simulink model "VirtualMotoTemplate"  (R2025b)
settings: Solver=daessc  StartTime=0  StopTime=2474  FixedStep=.001  RelTol=1e-2  EnableMultiTasking=on
StopFcn:
  | %toc
undefined symbols (not defined in the file): AccelOvrCmd, CtrlTcuInitGear, DecelOvrCmd, Disabled, DriverPreviewDist, EnblAccelOvr, EnblDecelCmd, EnblSteerCmd, EnvAbsPrs, EnvAirTemp, EnvGrvty, EnvNomFrictionScaling, EnvNominalGrade, EnvWindVelX, EnvWindVelY, EnvWindVelZ, FTP75, MotoFrmInert, MotoFrmLngth, MotoFrmMass, MotoLowrFrntFrkMass, MotoRearArmLngth, MotoRearArmMass, MotoUpprFrntFrkMass, RiderLkAhdPtDstGain, RiderMass, ScnAccTbl, ScnBrkTbl, ScnCRMaxLatAccel, ScnCRRadius, ScnDLCGateLongPos, ScnDLCLatRef, ScnDLCLatRefOffset, ScnDLCLongRefBpt, ScnDLCLongRefStartPos, ScnDLCVehicleWidth, ScnFHCounterDwellTime, ScnFHInitialDwellTime, ScnFHReturnTime, ScnFHRollRateZeroCross, ScnFHSteerAmp, ScnFHSteerSpeed, ScnISHandwheelRate, ScnISMaxHandwheelAng, ScnISMaxLatAccel, ScnISSteerHoldTime, ScnLongPosBpts, ScnLongVelRef, ScnOvalTrackl, ScnOvalTrackpdst, ScnOvalTrackr, ScnSDDwellTime, ScnSDSteerAmp, ScnSDSteerFreq, ScnSSFinalFreq, ScnSSSteerAmp, ScnSSSweepTime, ScnStartTime, ScnStrgAngTbl, ScnStrgTrqTbl ... (+10)
libraries: simulink x16, vehdynlibscenariocommon x9, sm_lib x6, autolibshared x4, nesl_utility x4, vehdynlibviscommon x3, sim3dgroundtruthsensorlib x2, vehdynlibdriver x2, sharedtransform x1, autolibutils x1, sim3dautolib x1, sim3dlib x1
(part 2 of 6)

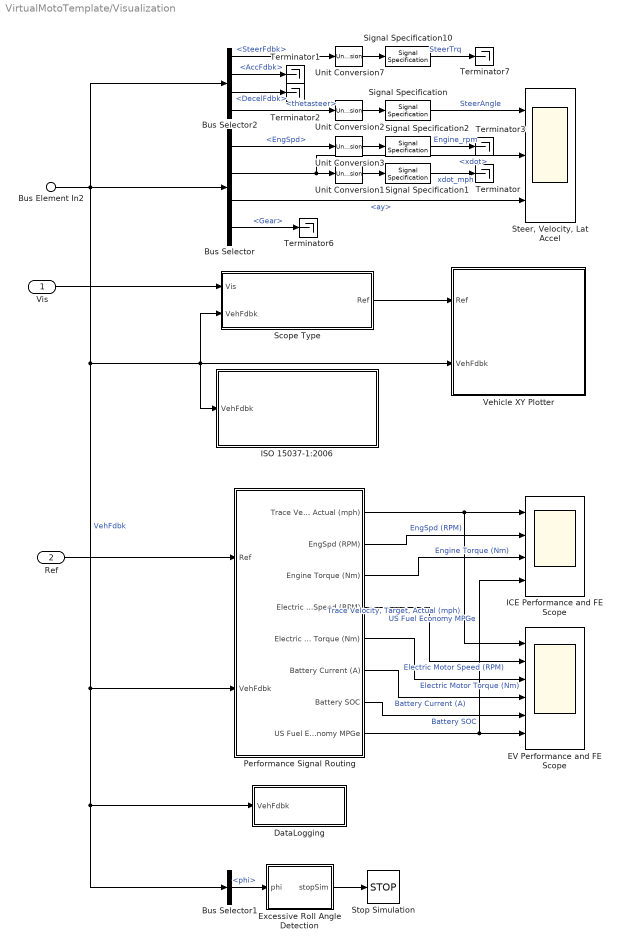
== system VirtualMotoTemplate/Visualization ==
  Vis : Inport
  Ref : Inport  Port=2
  Bus Element In2 : Inport  Port=3  PortName=VehFdbk
  Bus Selector : BusSelector  OutputSignals=Driveline.EngSpd,Body.BdyFrm.Cg.Vel.xdot,Body.BdyFrm.Cg.Acc.ay,Driveline.Gear
  Bus Selector1 : BusSelector  OutputSignals=Body.InertFrm.Cg.Ang.phi
  Bus Selector2 : BusSelector  OutputSignals=Rider.SteerFdbk,Rider.AccFdbk,Rider.DecelFdbk,Steer.Genrl.Ang.thetasteer
  DataLogging : Subsystem
  EV Performance and FE Scope : Scope  NumInputPorts=6
      settings: SampleTime=0.1  ActiveDisplayYMinimum=-0.55336  ActiveDisplayYMaximum=25.23635
  Excessive Roll Angle Detection : MATLAB Function  TreatAsAtomicUnit=on  SystemSampleTime=.1
  ICE Performance and FE Scope : Scope  NumInputPorts=4
      settings: SampleTime=0.1  ActiveDisplayYMinimum=-3.00968  ActiveDisplayYMaximum=25.77885
  ISO 15037-1:2006 : Subsystem  StopFcn=|  Variant=on  VariantControlMode=label  LabelModeActiveChoice=0  mask(ISO 15037-1:2006){Measurement=Disabled}
      | switch get_param(gcb,'Measurement')
      |     case 'Enabled'
      |        p=slproject.getCurrentProject;
      |        projectRoot=p.RootFolder;
      |        SySFolder=fullfile(projectRoot, 'System');
      |        Simulink.sdi.loadView([SySFolder filesep 'ISO15037_1_2006E.mldatx']);
      |        Simulink.sdi.view;
      | end
      mask prompts: Measurement "ISO Measurements"
      mask help: Enables display of ISO 15037-1:2006 standard measurement signals in the Simulation Data Inspector.
      mask init:
      | switch get_param(gcb,'Measurement')
      |     case 'Disabled'
      |         set_param(gcb,'OverrideUsingVariant','0')
      |     case 'Enabled'
      |        set_param(gcb,'OverrideUsingVariant','1')
      |     otherwise
      |        set_param(gcb,'OverrideUsingVariant','0')
      | end
      settings: AttributesFormatString=%<Measurement>
      mask Help: eval('vdynblkshelp(''iso15037'')');
      mask TypeOptions Measurement: Enabled | Disabled
      mask Callback Measurement:
      | switch get_param(gcb,'Measurement')
      |     case 'Disabled'
      |         set_param(gcb,'OverrideUsingVariant','0')
      |     case 'Enabled'
      |        set_param(gcb,'OverrideUsingVariant','1')
      |     otherwise
      |        set_param(gcb,'OverrideUsingVariant','0')
      | end
      mask Display: disp('ISO 15037-1:2006')
  Performance Signal Routing : Subsystem
  Scope Type : Subsystem  Variant=on  VariantControlMode=label  VariantControl=Variant1  LabelModeActiveChoice=0
  Signal Specification : SignalSpecification  Unit=deg
  Signal Specification1 : SignalSpecification  Unit=mph
  Signal Specification10 : SignalSpecification  Unit=N*m
  Signal Specification2 : SignalSpecification  Unit=rpm
  "Steer, Velocity, Lat Accel" : Scope  NumInputPorts=3
      settings: ActiveDisplayYMinimum=-4.93239  ActiveDisplayYMaximum=44.39148
  Stop Simulation : Stop
  Terminator{,1..3,6..7} (6 alike) : Terminator
  Unit Conversion{1..3,7} (4 alike) : UnitConversion
  Vehicle XY Plotter : Subsystem  Variant=on  VariantControlMode=label  VariantControl=Variant1  LabelModeActiveChoice=2
  wires:
  Signal Specification/1 -> "Steer, Velocity, Lat Accel"/1  "SteerAngle"
  Unit Conversion2/1 -> Signal Specification/1
  Vis/1 -> Scope Type/1("Vis ")
  Scope Type/1(" Ref") -> Vehicle XY Plotter/1("Ref ")
  Bus Selector/3 -> "Steer, Velocity, Lat Accel"/3  "<ay>"
  Bus Element In2/1 -> Bus Selector1/1, DataLogging/1(VehFdbk), Performance Signal Routing/2(VehFdbk), Scope Type/2("VehFdbk "), Vehicle XY Plotter/2("VehFdbk "), ISO 15037-1:2006/1(VehFdbk), Bus Selector2/1, Bus Selector/1  "VehFdbk"
  Bus Selector/2 -> Unit Conversion1/1, "Steer, Velocity, Lat Accel"/2  "<xdot>"
  Bus Selector2/2 -> Terminator1/1  "<AccFdbk>"
  Bus Selector2/3 -> Terminator2/1  "<DecelFdbk>"
  Bus Selector2/4 -> Unit Conversion2/1  "<thetasteer>"
  Unit Conversion1/1 -> Signal Specification1/1
  Unit Conversion3/1 -> Signal Specification2/1
  Bus Selector/1 -> Unit Conversion3/1  "<EngSpd>"
  Signal Specification2/1 -> Terminator3/1  "Engine_rpm"
  Signal Specification1/1 -> Terminator/1  "xdot_mph"
  Bus Selector/4 -> Terminator6/1  "<Gear>"
  Bus Selector2/1 -> Unit Conversion7/1  "<SteerFdbk>"
  Signal Specification10/1 -> Terminator7/1  "SteerTrq"
  Unit Conversion7/1 -> Signal Specification10/1
  Performance Signal Routing/1("Trace Velocity, Target, Actual (mph)") -> EV Performance and FE Scope/1, ICE Performance and FE Scope/1  "Trace Velocity, Target, Actual (mph)"
  Performance Signal Routing/8(US Fuel Economy MPGe) -> ICE Performance and FE Scope/4, EV Performance and FE Scope/6  "US Fuel Economy MPGe"
  Ref/1 -> Performance Signal Routing/1(Ref)
  Performance Signal Routing/2(EngSpd (RPM)) -> ICE Performance and FE Scope/2  "EngSpd (RPM)"
  Performance Signal Routing/3(Engine Torque (Nm)) -> ICE Performance and FE Scope/3  "Engine Torque (Nm)"
  Performance Signal Routing/4(Electric Motor Speed (RPM)) -> EV Performance and FE Scope/2  "Electric Motor Speed (RPM)"
  Performance Signal Routing/5(Electric Motor Torque (Nm)) -> EV Performance and FE Scope/3  "Electric Motor Torque (Nm)"
  Performance Signal Routing/6(Battery Current (A)) -> EV Performance and FE Scope/4  "Battery Current (A)"
  Performance Signal Routing/7(Battery SOC) -> EV Performance and FE Scope/5  "Battery SOC"
  Bus Selector1/1 -> Excessive Roll Angle Detection/1(phi)  "<phi>"
  Excessive Roll Angle Detection/1(stopSim) -> Stop Simulation/1

== system VirtualMotoTemplate/Controllers/Battery Management System (BMS) ==
  note: 1) Add Subsystem or Model blocks as valid variant choices.
      | 2) You cannot connect blocks at this level. At simulation, connectivity is automatically
      | determined, based on the active variant and port name matching.
  BMSSensors : Inport
  BMSController : ModelReference  ModelNameDialog=BMSController.slx  SimulationMode=Normal  VariantControl=BMSController  ModelReferenceVersion=11.0
  NoBMS : Subsystem  VariantControl=NoBMS  ReferencedSubsystem=NoBMS
  BMSInfo : Outport
  BMSCmd : Outport  Port=2

== system VirtualMotoTemplate/Controllers/Brake Control Unit (BCU) ==
  note: 1) Add Subsystem or Model blocks as valid variant choices.
      | 2) You cannot connect blocks at this level. At simulation, connectivity is automatically
      | determined, based on the active variant and port name matching.
  DecelFdbk : Inport  PortDimensions=2
  Omega : Inport  Port=2
  Accel : Inport  Port=3
  BangBangABS : ModelReference  ModelNameDialog=BangBangABS  SimulationMode=Normal  VariantControl=BangBangABS  ModelReferenceVersion=4.10
  FiveStateABSforMotorcycle : ModelReference  ModelNameDialog=FiveStateABSforMotorcycle  SimulationMode=Normal  VariantControl=FiveStateABSforMotorcycle  ModelReferenceVersion=4.8
  OpenLoopController : ModelReference  ModelNameDialog=OpenLoopController  SimulationMode=Normal  VariantControl=OpenLoopController  ModelReferenceVersion=4.2
  BrkPrsCmd : Outport  VectorParamsAs1DForOutWhenUnconnected=off
  ABSFlag : Outport  Port=2  VectorParamsAs1DForOutWhenUnconnected=off

== system VirtualMotoTemplate/Controllers/Engine Control Unit (ECU) ==
  note: 1) Add Subsystem or Model blocks as valid variant choices.
      | 2) You cannot connect blocks at this level. At simulation, connectivity is automatically
      | determined, based on the active variant and port name matching.
  TrqCmd : Inport
  EngSpd : Inport  Port=2
  ABSFlag : Inport  Port=3
  MotoNoEngineController : Subsystem  VariantControl=MotoNoEngineController  ReferencedSubsystem=MotoNoEngineController
  MotoSimpleECU : Subsystem  VariantControl=MotoSimpleECU  ReferencedSubsystem=MotoSimpleECU
  EngTrqCmd : Outport

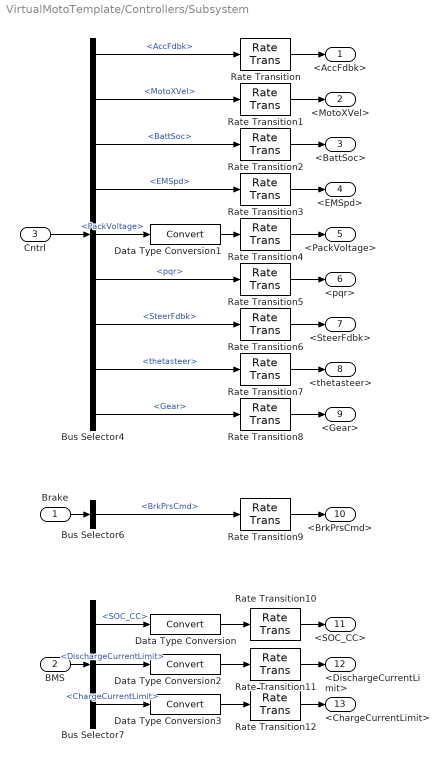
== system VirtualMotoTemplate/Controllers/Subsystem ==
  Brake : Inport
  BMS : Inport  Port=2
  Cntrl : Inport  Port=3
  Bus Selector4 : BusSelector  OutputSignals=Rider.AccFdbk,MotoXVel,Battery.BattSoc,Trans.EMSpd,Battery.BMSSensors.PackVoltage,IMU.pqr,Rider.SteerFdbk,Steering.Genrl.Ang.thetasteer,Trans.Gear
  Bus Selector6 : BusSelector  OutputSignals=BrkPrsCmd
  Bus Selector7 : BusSelector  OutputSignals=BMSInfo.SOC.SOC_CC,BMSCmd.CurrentLimitsBus.DischargeCurrentLimit,BMSCmd.CurrentLimitsBus.ChargeCurrentLimit
  Data Type Conversion{,1..3} (4 alike) : DataTypeConversion  SaturateOnIntegerOverflow=off  RndMeth=Floor
  Rate Transition{,1..12} (13 alike) : RateTransition  Deterministic=off
  <AccFdbk> : Outport
  <MotoXVel> : Outport  Port=2
  <BattSoc> : Outport  Port=3
  <EMSpd> : Outport  Port=4
  <PackVoltage> : Outport  Port=5
  <pqr> : Outport  Port=6
  <SteerFdbk> : Outport  Port=7
  <thetasteer> : Outport  Port=8
  <Gear> : Outport  Port=9
  <BrkPrsCmd> : Outport  Port=10
  <SOC_CC> : Outport  Port=11
  <DischargeCurrentLimit> : Outport  Port=12
  <ChargeCurrentLimit> : Outport  Port=13
  wires:
  Bus Selector4/3 -> Rate Transition2/1  "<BattSoc>"
  Cntrl/1 -> Bus Selector4/1
  Bus Selector4/2 -> Rate Transition1/1  "<MotoXVel>"
  Bus Selector4/6 -> Rate Transition5/1  "<pqr>"
  Bus Selector7/1 -> Data Type Conversion/1  "<SOC_CC>"
  Bus Selector7/2 -> Data Type Conversion2/1  "<DischargeCurrentLimit>"
  Bus Selector4/8 -> Rate Transition7/1  "<thetasteer>"
  Bus Selector4/1 -> Rate Transition/1  "<AccFdbk>"
  BMS/1 -> Bus Selector7/1
  Bus Selector7/3 -> Data Type Conversion3/1  "<ChargeCurrentLimit>"
  Bus Selector4/4 -> Rate Transition3/1  "<EMSpd>"
  Brake/1 -> Bus Selector6/1
  Bus Selector4/9 -> Rate Transition8/1  "<Gear>"
  Bus Selector4/7 -> Rate Transition6/1  "<SteerFdbk>"
  Bus Selector6/1 -> Rate Transition9/1  "<BrkPrsCmd>"
  Bus Selector4/5 -> Data Type Conversion1/1  "<PackVoltage>"
  Data Type Conversion1/1 -> Rate Transition4/1
  Data Type Conversion/1 -> Rate Transition10/1
  Data Type Conversion2/1 -> Rate Transition11/1
  Data Type Conversion3/1 -> Rate Transition12/1
  Rate Transition/1 -> <AccFdbk>/1
  Rate Transition1/1 -> <MotoXVel>/1
  Rate Transition2/1 -> <BattSoc>/1
  Rate Transition3/1 -> <EMSpd>/1
  Rate Transition4/1 -> <PackVoltage>/1
  Rate Transition5/1 -> <pqr>/1
  Rate Transition6/1 -> <SteerFdbk>/1
  Rate Transition7/1 -> <thetasteer>/1
  Rate Transition8/1 -> <Gear>/1
  Rate Transition9/1 -> <BrkPrsCmd>/1
  Rate Transition10/1 -> <SOC_CC>/1
  Rate Transition11/1 -> <DischargeCurrentLimit>/1
  Rate Transition12/1 -> <ChargeCurrentLimit>/1

== system VirtualMotoTemplate/Controllers/Subsystem1 ==
  VCU : Inport
  CntrlRx : Inport  Port=2
  Brake : Inport  Port=3
  Bus Selector2 : BusSelector  OutputSignals=Engine.EngineInfo.EngSpd
  Bus Selector4 : BusSelector  OutputSignals=EngTrqCmd
  Bus Selector6 : BusSelector  OutputSignals=ABSFlag
  Rate Transition : RateTransition  Deterministic=off
  Rate Transition1 : RateTransition  Deterministic=off
  Rate Transition2 : RateTransition  Deterministic=off
  <EngTrqCmd> : Outport
  <EngSpd> : Outport  Port=2
  <ABSFlag> : Outport  Port=3
  wires:
  Bus Selector2/1 -> Rate Transition2/1  "<EngSpd>"
  Bus Selector4/1 -> Rate Transition/1  "<EngTrqCmd>"
  VCU/1 -> Bus Selector4/1
  Bus Selector6/1 -> Rate Transition1/1  "<ABSFlag>"
  Brake/1 -> Bus Selector6/1
  CntrlRx/1 -> Bus Selector2/1
  Rate Transition/1 -> <EngTrqCmd>/1
  Rate Transition1/1 -> <ABSFlag>/1
  Rate Transition2/1 -> <EngSpd>/1

== system VirtualMotoTemplate/Controllers/Subsystem2 ==
  Brake : Inport
  CntrlRx : Inport  Port=2
  Bus Selector1 : BusSelector  OutputSignals=Rider.AccFdbk,Rider.DecelFdbk,Rider.GearFdbk,Engine.EngineInfo.EngSpd,Wheels.FrontTire.Omega,Wheels.RearTire.Omega
  Bus Selector5 : BusSelector  OutputSignals=ABSFlag
  Ground : Ground
  Ground1 : Ground
  Mux : Mux  Inputs=2
  Rate Transition{1..4,6..8} (7 alike) : RateTransition  Deterministic=off
  Rate Transition5 : RateTransition  Commented=through  Deterministic=off
  Signal Specification : SignalSpecification  Commented=through  Unit=rpm
  Unit Conversion : UnitConversion
  <ABSFlag> : Outport
  <AccFdbk> : Outport  Port=2
  <DecelFdbk> : Outport  Port=3
  <GearFdbk> : Outport  Port=4
  <EngSpd> : Outport  Port=5
  <Omega> : Outport  Port=6
  UpReq : Outport  Port=7
  DnReq : Outport  Port=8
  wires:
  Bus Selector1/6 -> Mux/2  "<Omega>"
  Brake/1 -> Bus Selector5/1
  Bus Selector1/4 -> Unit Conversion/1  "<EngSpd>"
  Bus Selector1/1 -> Rate Transition2/1  "<AccFdbk>"
  Bus Selector1/2 -> Rate Transition3/1  "<DecelFdbk>"
  Bus Selector1/3 -> Rate Transition4/1  "<GearFdbk>"
  CntrlRx/1 -> Bus Selector1/1
  Bus Selector5/1 -> Rate Transition1/1  "<ABSFlag>"
  Rate Transition8/1 -> DnReq/1
  Rate Transition7/1 -> UpReq/1
  Ground1/1 -> Rate Transition8/1
  Ground/1 -> Rate Transition7/1
  Rate Transition1/1 -> <ABSFlag>/1
  Rate Transition2/1 -> <AccFdbk>/1
  Rate Transition3/1 -> <DecelFdbk>/1
  Rate Transition4/1 -> <GearFdbk>/1
  Rate Transition5/1 -> <EngSpd>/1
  Rate Transition6/1 -> <Omega>/1
  Bus Selector1/5 -> Mux/1  "<Omega>"
  Mux/1 -> Rate Transition6/1
  Unit Conversion/1 -> Signal Specification/1
  Signal Specification/1 -> Rate Transition5/1  "EngSpd"

== system VirtualMotoTemplate/Controllers/Subsystem3 ==
  CntrlRx : Inport
  Bus Selector : BusSelector  OutputSignals=Rider.DecelFdbk,Wheels.FrontTire.Omega,Wheels.RearTire.Omega,IMU.Acc
  Mux : Mux  Inputs=2
  Rate Transition : RateTransition  Deterministic=off
  Rate Transition1 : RateTransition  Deterministic=off
  Rate Transition2 : RateTransition  Deterministic=off
  Unary Minus : UnaryMinus
  <DecelFdbk> : Outport
  Omega : Outport  Port=2
  <Acc> : Outport  Port=3
  wires:
  Unary Minus/1 -> Rate Transition1/1
  Mux/1 -> Unary Minus/1
  Bus Selector/1 -> Rate Transition/1  "<DecelFdbk>"
  Bus Selector/4 -> Rate Transition2/1  "<Acc>"
  CntrlRx/1 -> Bus Selector/1
  Rate Transition/1 -> <DecelFdbk>/1
  Rate Transition1/1 -> Omega/1
  Rate Transition2/1 -> <Acc>/1
  Bus Selector/3 -> Mux/2  "<Omega>"
  Bus Selector/2 -> Mux/1  "<Omega>"

== system VirtualMotoTemplate/Controllers/Subsystem4 ==
  BrkPrsCmd : Inport
  ABSFlag : Inport  Port=2
  Bus Creator2 : BusCreator  Inputs=2
  Data Type Conversion : DataTypeConversion  OutDataTypeStr=double  SaturateOnIntegerOverflow=off  RndMeth=Floor
  Data Type Conversion1 : DataTypeConversion  OutDataTypeStr=boolean  SaturateOnIntegerOverflow=off  RndMeth=Floor
  First Order Hold : FirstOrderHold  ErrorTolerance=0.1  AllowContinuousInput=on
  First Order Hold1 : FirstOrderHold  ErrorTolerance=1  AllowContinuousInput=on
  Brake : Outport
  wires:
  First Order Hold/1 -> Bus Creator2/2  "BrkPrsCmd"
  Data Type Conversion1/1 -> Bus Creator2/1  "ABSFlag"
  Bus Creator2/1 -> Brake/1  "Brake"
  BrkPrsCmd/1 -> First Order Hold/1
  ABSFlag/1 -> Data Type Conversion/1
  Data Type Conversion/1 -> First Order Hold1/1
  First Order Hold1/1 -> Data Type Conversion1/1

== system VirtualMotoTemplate/Controllers/Transmission Control Unit (TCU) ==
  ABSFlag : Inport  PortDimensions=2
  Accel : Inport  Port=2
  BrkCmd : Inport  Port=3  PortDimensions=2
  GearReq : Inport  Port=4
  EngSpd : Inport  Port=5
  Omega : Inport  Port=6  Unit=rad/s
  UpReq : Inport  Port=7
  DownReq : Inport  Port=8  Unit=rad/s
  PRNDLController : ModelReference  ModelNameDialog=PRNDLController  SimulationMode=Normal  VariantControl=PRNDLController  ModelReferenceVersion=4.12
  Paddles : ModelReference  ModelNameDialog=Paddles  SimulationMode=Normal  VariantControl=Paddles  ModelReferenceVersion=4.3
  RiderPassThrough : ModelReference  ModelNameDialog=RiderPassThrough  SimulationMode=Normal  VariantControl=RiderPassThrough  ModelReferenceVersion=4.3
  TransmissionController : ModelReference  ModelNameDialog=TransmissionController  SimulationMode=Normal  VariantControl=TransmissionController  ModelReferenceVersion=4.4
  " Gear" : Outport  VectorParamsAs1DForOutWhenUnconnected=off

== system VirtualMotoTemplate/Controllers/Vehicle Control Unit (VCU) ==
  AccelPdl : Inport
  VehSpdFdbk : Inport  Port=2
  BattSoc : Inport  Port=3
  EMSpd : Inport  Port=4
  BattPackVolt : Inport  Port=5
  pqr : Inport  Port=6
  SteerCmd : Inport  Port=7
  SteerWhlAng : Inport  Port=8
  TransGear : Inport  Port=9
  BcuBrkPrsCmd : Inport  Port=10
  BMSSOC : Inport  Port=11
  BMSDischrgCurrLmt : Inport  Port=12
  BMSChrgCurrLmt : Inport  Port=13
  EMotoPowertrainController : ModelReference  ModelNameDialog=EMotoPowertrainController  VariantControl=EMotoPowertrainController  ModelReferenceVersion=11.2
  EMotoPowertrainControllerBMS : ModelReference  ModelNameDialog=EMotoPowertrainControllerBMS.slx  VariantControl=EMotoPowertrainControllerBMS  ModelReferenceVersion=6.15
  NoVCU : ModelReference  ModelNameDialog=NoVCU  SimulationMode=Normal  VariantControl=NoVCU  ModelReferenceVersion=4.4
  EngTrqCmd : Outport  VectorParamsAs1DForOutWhenUnconnected=off
  EMTrqCmd : Outport  Port=2  VectorParamsAs1DForOutWhenUnconnected=off
  VcuBrkPrsCmd : Outport  Port=3  VectorParamsAs1DForOutWhenUnconnected=off

== system VirtualMotoTemplate/Environment/Estimated Grade ==
  Gnd : Inport
  Atan : Trigonometry  Operator=atan
  Bus Selector : BusSelector  OutputSignals=z  OutputAsBus=on
  Bus to Vector : BusToVector
  Constant Grade : Constant  Value=EnvNominalGrade  SampleTime=-1
  Constant1 : Constant  Value=MotoFrmLngth  SampleTime=-1
  Divide : Product  Inputs=*/
  Grade Source : ManualSwitch  CurrentSetting=0
  Selector : Selector  InputPortWidth=2  IndexOptions=Index vector (dialog)  Indices=[1]  OutputSizes=1
  Selector1 : Selector  InputPortWidth=2  IndexOptions=Index vector (dialog)  Indices=[2]  OutputSizes=1
  Signal Specification : SignalSpecification  Unit=rad
  Signal Specification1 : SignalSpecification  Unit=deg
  Signal Specification2 : SignalSpecification  Unit=deg
  Subtract : Sum  Inputs=+-
  Unit Conversion : UnitConversion
  Grade : Outport  PortDimensions=1
  wires:
  Divide/1 -> Atan/1
  Bus Selector/1 -> Bus to Vector/1
  Selector/1 -> Subtract/1
  Signal Specification/1 -> Unit Conversion/1
  Constant1/1 -> Divide/2
  Selector1/1 -> Subtract/2
  Subtract/1 -> Divide/1
  Atan/1 -> Signal Specification/1
  Grade Source/1 -> Grade/1  "Grade"
  Gnd/1 -> Bus Selector/1
  Bus to Vector/1 -> Selector1/1, Selector/1
  Constant Grade/1 -> Signal Specification2/1
  Signal Specification2/1 -> Grade Source/2
  Unit Conversion/1 -> Signal Specification1/1
  Signal Specification1/1 -> Grade Source/1  "Grade"

== system VirtualMotoTemplate/Environment/Friction ==
  MotoFdbk : Inport
  Constant Friction : Subsystem  VariantControl=Constant Friction
  Varying Friction : Subsystem  VariantControl=Varying Friction
  FricCoeffLambda : Outport

== system VirtualMotoTemplate/Environment/Ground Feedback ==
  Friction : Inport
  WheelFdbk : Inport  Port=2
  3D Engine : Subsystem  VariantControl=1
  Constant : Subsystem  VariantControl=0
  Ground : Outport  VectorParamsAs1DForOutWhenUnconnected=off

== system VirtualMotoTemplate/Motorcycle Vehicle/Body, Steer, Suspension, Wheels ==
  Env : Inport
  Driveline : Inport  Port=2
  Rider : Inport  Port=3
  "Body, Steer, Suspension, Wheels" : Subsystem  Variant=on  VariantChoicesSpecifier={'In_Plane_Model', 'Out_of_Plane_Model'}  VariantControlMode=label  VariantControl=Choice  LabelModeActiveChoice=In_Plane_Model
      mask Display: disp('Body,Steer,Suspension,Wheels');
  Chassis Input : Subsystem
  Chassis Output : Subsystem
  MotoFdbk : Outport
  WheelsFdbk : Outport  Port=2
  wires:
  Chassis Input/1(Wind) -> "Body, Steer, Suspension, Wheels"/1(WindXYZ)
  "Body, Steer, Suspension, Wheels"/1(Moto) -> Chassis Output/1(Moto)
  Chassis Input/2(BrkPrs) -> "Body, Steer, Suspension, Wheels"/2(BrkPrs)
  "Body, Steer, Suspension, Wheels"/2(Wheels) -> Chassis Output/2(Wheels)
  Chassis Input/4(MDrvArmR) -> "Body, Steer, Suspension, Wheels"/4(MDrvArmR)
  Chassis Input/6(ScaleFactrs) -> "Body, Steer, Suspension, Wheels"/6(ScaleFactrs)
  Chassis Input/3(MDrvSprtR) -> "Body, Steer, Suspension, Wheels"/3(MDrvSprtR)
  Chassis Input/5(MDrvFrm) -> "Body, Steer, Suspension, Wheels"/5(MDrvFrm)
  Env/1 -> Chassis Input/1(Env)
  Driveline/1 -> Chassis Input/2(Driveline)
  Chassis Output/2(WheelsFdbk) -> WheelsFdbk/1
  Chassis Output/1(MotoFdbk) -> MotoFdbk/1
  Chassis Input/7(SteerCmd) -> "Body, Steer, Suspension, Wheels"/7(SteerCmd)
  Rider/1 -> Chassis Input/3(Rider)

== system VirtualMotoTemplate/Motorcycle Vehicle/Control Feedback ==
  MotoFdbk : Inport
  Rider : Inport  Port=2
  Engine : Inport  Port=3
  Battery : Inport  Port=4
  EM : Inport  Port=5
  Env : Inport  Port=6
  Driveline : Inport  Port=7
  Wheels : Inport  Port=8
  Bus Selector1 : BusSelector  OutputSignals=Steer
  Bus Selector2 : BusSelector  OutputSignals=Susp
  Bus Selector7 : BusSelector  OutputSignals=BattSoc,BattVolt,BattCurr,BattPwr,BMSSensors  OutputAsBus=on
  Bus Selector8 : BusSelector  OutputSignals=Frame.BdyFrm.Cg.Vel.xdot  OutputAsBus=on
  Bus Selector9 : BusSelector  OutputSignals=EMTrq,EMPwrElec  OutputAsBus=on
  Variant Subsystem : Subsystem  Variant=on  VariantControlMode=label  LabelModeActiveChoice=No_IMU_Sensor
  Bus Element Out : Outport  PortName=CntrlRx  Element=MotoXVel
  Bus Element Out1 : Outport  PortName=CntrlRx  Element=Rider
  Bus Element Out2 : Outport  PortName=CntrlRx  Element=Engine
  Bus Element Out3 : Outport  PortName=CntrlRx  Element=Trans
  Bus Element Out4 : Outport  PortName=CntrlRx  Element=Battery
  Bus Element Out5 : Outport  PortName=CntrlRx  Element=EM
  Bus Element Out7 : Outport  PortName=CntrlRx  Element=Wheels
  Bus Element Out8 : Outport  PortName=CntrlRx  Element=IMU
  Bus Element Out9 : Outport  PortName=CntrlRx  Element=Env
  Bus Element Out10 : Outport  PortName=CntrlRx  Element=Steering
  Bus Element Out11 : Outport  PortName=CntrlRx  Element=Suspension
  wires:
  Bus Selector2/1 -> Bus Element Out11/1  "<Susp>"
  Wheels/1 -> Bus Element Out7/1
  Bus Selector7/1 -> Bus Element Out4/1  "Battery"
  Bus Selector8/1 -> Bus Element Out/1  "Moto"
  Bus Selector9/1 -> Bus Element Out5/1  "EM"
  Engine/1 -> Bus Element Out2/1
  Battery/1 -> Bus Selector7/1
  EM/1 -> Bus Selector9/1
  MotoFdbk/1 -> Variant Subsystem/1(MotoFdbk), Bus Selector1/1, Bus Selector2/1, Bus Selector8/1  "Moto"
  Variant Subsystem/1(IMU) -> Bus Element Out8/1  "IMU"
  Rider/1 -> Bus Element Out1/1  "Rider"
  Env/1 -> Bus Element Out9/1  "Env"
  Bus Selector1/1 -> Bus Element Out10/1  "<Steer>"
  Driveline/1 -> Bus Element Out3/1

== system VirtualMotoTemplate/Motorcycle Vehicle/Hand Levers and Pedals ==
  Rider : Inport
  Driveline : Inport  Port=2
  Hand Levers and Pedals : Subsystem
  Pedal Cluster Input : Subsystem
  Pedal Cluster Output : Subsystem
  OperatorFdbk : Outport
  wires:
  Hand Levers and Pedals/4(GearFdbk) -> Pedal Cluster Output/4(GearFdbk)
  Hand Levers and Pedals/2(AccFdbk) -> Pedal Cluster Output/2(AccFdbk)
  Pedal Cluster Input/5(BrkPrs) -> Hand Levers and Pedals/5(BrkPrs)
  Pedal Cluster Input/1(SteerCmd) -> Hand Levers and Pedals/1(SteerCmd)
  Pedal Cluster Input/6(StrWhlTrq) -> Hand Levers and Pedals/6(StrWhlTrq)
  Pedal Cluster Input/3(DecelCmd) -> Hand Levers and Pedals/3(DecelCmd)
  Hand Levers and Pedals/3(DecelFdbk) -> Pedal Cluster Output/3(DecelFdbk)
  Pedal Cluster Input/2(AccelCmd) -> Hand Levers and Pedals/2(AccCmd)
  Pedal Cluster Input/4(GearCmd) -> Hand Levers and Pedals/4(GearCmd)
  Rider/1 -> Pedal Cluster Input/1(Rider)
  Hand Levers and Pedals/1(SteerFdbk) -> Pedal Cluster Output/1(SteerFdbk)
  Pedal Cluster Output/1(OperatorFdbk) -> OperatorFdbk/1
  Driveline/1 -> Pedal Cluster Input/2(Driveline)

== system VirtualMotoTemplate/Motorcycle Vehicle/Propulsion System ==
  Cntrl : Inport
  Driveline : Inport  Port=2
  Env : Inport  Port=3
  Actuators : Subsystem  Variant=on  VariantChoicesSpecifier={'MotoMappedEngine', 'MotoElectricalSystem', 'MotoSimpleEngine'}  VariantControlMode=label  LabelModeActiveChoice=MotoSimpleEngine
  Electrical System Input : Subsystem
  Engine Input : Subsystem
  EngineFdbk : Outport
  BatteryFdbk : Outport  Port=2
  ElecMachineFdbk : Outport  Port=3
  wires:
  Actuators/1(Eng) -> EngineFdbk/1
  Engine Input/2(EngSpd) -> Actuators/2(EngSpd)
  Cntrl/1 -> Electrical System Input/1(Cntrl), Engine Input/1(Cntrl)
  Engine Input/1(EngTrqCmd) -> Actuators/1(TrqCmd)
  Driveline/1 -> Electrical System Input/2(Driveline), Engine Input/2(Driveline)
  Actuators/2(Battery) -> BatteryFdbk/1
  Actuators/3(ElecMachine) -> ElecMachineFdbk/1
  Electrical System Input/1(EMTrqCmd) -> Actuators/3(EMTrqCmd)
  Electrical System Input/2(EMSpd) -> Actuators/4(EMSpd)
  Electrical System Input/3(AmbTemp) -> Actuators/5(AmbTemp)
  Env/1 -> Electrical System Input/3(Env)

== system VirtualMotoTemplate/Motorcycle Vehicle/Transmission, Driveline and Brakes ==
  Cntrl : Inport
  EngTrqCmd : Inport  Port=2
  Wheels : Inport  Port=3
  Moto : Inport  Port=4
  EMTrqCmd : Inport  Port=5
  Brake Hydraulics : Subsystem
  Driveline Input : Subsystem
  Driveline Output : Subsystem
  Transmission and Driveline : Subsystem
  Driveline : Outport
  wires:
  Transmission and Driveline/2(Gear) -> Driveline Output/2(Gear)
  Driveline Input/6(MBrkR.) -> Transmission and Driveline/6(MBrkR)
  Driveline Input/3(FCpR.) -> Transmission and Driveline/3(FCpR)
  Transmission and Driveline/1(EngSpd) -> Driveline Output/1(EngSpd)
  Driveline Input/1(EngTrq) -> Transmission and Driveline/1(EngTrq)
  Driveline Input/4(ThetaFrm.) -> Transmission and Driveline/4(ThetaFrm)
  Transmission and Driveline/3(Info) -> Driveline Output/3(Info)
  Driveline Input/2(GearCmd) -> Transmission and Driveline/2(GearCmd)
  Driveline Input/7(AngAWhlR.) -> Transmission and Driveline/7(AngAWhlR)
  Driveline Input/5(ThetaArmR.) -> Transmission and Driveline/5(ThetaArmR)
  Cntrl/1 -> Driveline Input/1(Cntrl)
  EngTrqCmd/1 -> Driveline Input/2(EngTrqCmd)
  Wheels/1 -> Driveline Input/3(Wheels)
  Moto/1 -> Driveline Input/4(Moto)
  Driveline Output/1(Driveline) -> Driveline/1  "Driveline"
  Driveline Input/8(EMTrq) -> Transmission and Driveline/8(EMTrq)
  Transmission and Driveline/4(EMSpd) -> Driveline Output/4(EMSpd)
  EMTrqCmd/1 -> Driveline Input/5(EMTrqCmd)
  Driveline Input/9(BrkPrsCmd) -> Brake Hydraulics/1(BrkPrsCmd)
  Brake Hydraulics/1(BrkPrs) -> Driveline Output/5(BrkPrs)

== system VirtualMotoTemplate/Reference Generator for Motorcycle/3D Engine ==
  note: 1) Add Subsystem or Model blocks as valid variant choices.
      | 2) You cannot connect blocks at this level. At simulation, connectivity is automatically
      | determined, based on the active variant and port name matching.
  MotoFdbk : Inport
  3D Engine : Subsystem  VariantControl=Enabled
  3D Engine Disabled : Subsystem  VariantControl=Disabled

== system VirtualMotoTemplate/Reference Generator for Motorcycle/Reference Generator ==
  "MotoFdbk " : Inport
  Constant Radius : vehdynlibscenariocommon/Constant Radius  VariantControl=Constant Radius  t_start=t_start  xdot_r=xdot_r  xdotUnit=mph  R=R  X_o=X_o  Y_o=Y_o  psi_o=psi_o  vehW=6  ay_max=cr_ay_max  steerDir=off  ay_stop=off  use3DCones=off  aMode=2
  Constant Radius RCP : vehdynlibscenariocommon/Constant Radius  VariantControl=Constant Radius RCP  t_start=t_start  xdot_r=xdot_r  xdotUnit=mph  R=R  X_o=X_o  Y_o=Y_o  psi_o=psi_o  vehW=6  ay_max=cr_ay_max  steerDir=off  ay_stop=off  use3DCones=off  aMode=2
  Double Lane Change : Subsystem  VariantControl=Double Lane Change
  Drive Cycle : Subsystem  VariantControl=Drive Cycle
  Fishhook : Subsystem  VariantControl=Fishhook
  Increasing Steer : Subsystem  VariantControl=Increasing Steer
  Longitudinal Maneuver Tracking : Subsystem  VariantControl=Longitudinal Maneuver Tracking
  Manual Maneuver Design : Subsystem  VariantControl=Manual Maneuver Design
  Moto Target Trajectory : vehdynlibscenariocommon/Moto Target Trajectory  VariantControl=Moto Target Trajectory  t_start=t_start  xdot_r=xdot_r  xdotUnit=mph  R=R  X_o=X_o  Y_o=Y_o  psi_o=psi_o  vehW=6  ay_max=cr_ay_max  steerDir=off  ay_stop=off  use3DCones=off  aMode=2  engine3D=0  manOverride=0  prevType=0  manType=Oval Track  Trajl=Trajl  Trajr=Trajr  Trajpointdist=Trajpointdist  TrajDataSource=Variable  TrajDatFileCSV=TrajDatFileCSV  TrajDatFile=TrajDatFile  CoordinateX=CoordinateX  CoordinateY=CoordinateY
  Sine with Dwell : Subsystem  VariantControl=Sine with Dwell
  Swept Sine : Subsystem  VariantControl=Swept Sine
  WOT : Subsystem  VariantControl=WOT
  " Vis" : Outport  VectorParamsAs1DForOutWhenUnconnected=off
  " Ref" : Outport  Port=2  VectorParamsAs1DForOutWhenUnconnected=off
  " Fdbk" : Outport  Port=3  VectorParamsAs1DForOutWhenUnconnected=off

== system VirtualMotoTemplate/Reference Generator for Motorcycle/Reference Router ==
  note: 1) Add Subsystem or Model blocks as valid variant choices.
      | 2) You cannot connect blocks at this level. At simulation, connectivity is automatically
      | determined, based on the active variant and port name matching.
  VisIn : Inport
  RefIn : Inport  Port=2
  FdbkIn : Inport  Port=3
  Maneuver Tracking : Subsystem  VariantControl=Maneuver Tracking
  Steering Command Override : Subsystem  VariantControl=Steering Command Override
  Steering and Accel and Brk Command Override : Subsystem  VariantControl=Steering and Accel and Brk Command Override
  Vis : Outport
  Ref : Outport  Port=2
  Fdbk : Outport  Port=3

== system VirtualMotoTemplate/Rider Commands/Rider Commands ==
  MotoRef : Inport
  MotoFdbk : Inport  Port=2
  Env : Inport  Port=3
  GearCmd : Inport  Port=4
  Longitudinal Rider : Subsystem  VariantControl=driverType==1
  Open Loop : Subsystem  VariantControl=driverType==2
  Predictive Rider : Subsystem  VariantControl=driverType==4
  Predictive Stanley Rider : Subsystem  VariantControl=driverType==3
  Roll angle control : Subsystem  VariantControl=driverType==6
  Target trajectory following - Look ahead point : Subsystem  VariantControl=driverType==5
  " Rider" : Outport  VectorParamsAs1DForOutWhenUnconnected=off

== system VirtualMotoTemplate/Rider Commands/Torque Control ==
  note: 1) Add Subsystem or Model blocks as valid variant choices.
      | 2) You cannot connect blocks at this level. At simulation, connectivity is automatically
      | determined, based on the active variant and port name matching.
  MotoRef : Inport
  MotoFdbk : Inport  Port=2
  RiderInput : Inport  Port=3
  AngleToTorque : Subsystem  VariantControl=TorqueControlType == 1  mask{DbWdth=0.05, StrRng=pi/4}
      mask prompts: DbWdth "Steering deadband width, DbWdth [rad]:"; StrRng "Steering angle limit, StrRng [rad]"
  Look ahead point model : Subsystem  VariantControl=TorqueControlType == 3
  NoTorqueControl : Subsystem  VariantControl=TorqueControlType == 2
  PID Control : Subsystem  VariantControl=TorqueControlType == 4
  Rider : Outport

== system VirtualMotoTemplate/Visualization/DataLogging ==
  VehFdbk : Inport
  Bus Selector : BusSelector  OutputSignals=Rider.SteerFdbk
  Terminator : Terminator
  wires:
  VehFdbk/1 -> Bus Selector/1
  Bus Selector/1 -> Terminator/1  "<SteerFdbk>"

== system VirtualMotoTemplate/Visualization/ISO 15037-1:2006 ==
  VehFdbk : Inport
  Disabled : Subsystem  VariantControl=0
  Enabled : Subsystem  VariantControl=1

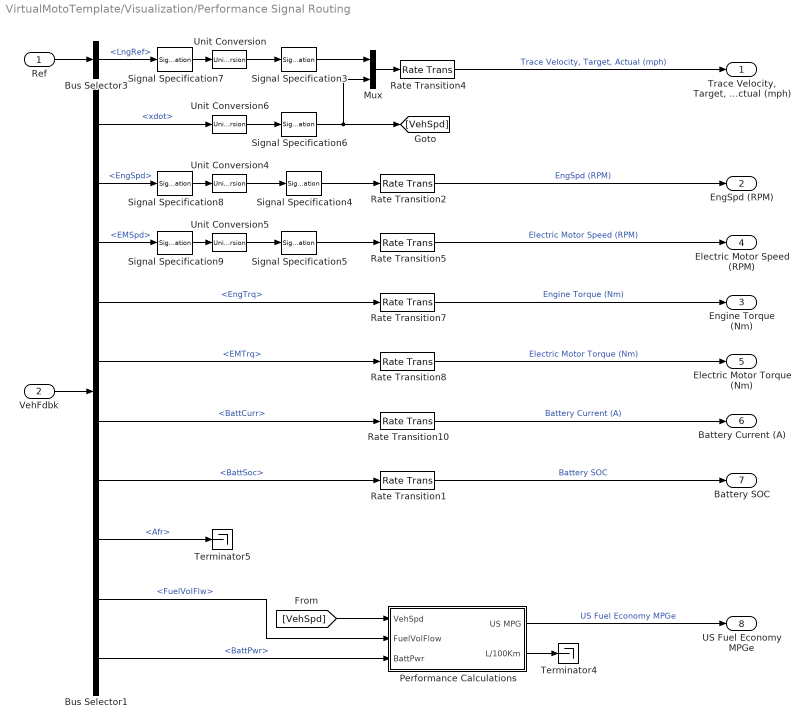
== system VirtualMotoTemplate/Visualization/Performance Signal Routing ==
  Ref : Inport
  VehFdbk : Inport  Port=2
  Bus Selector1 : BusSelector  OutputSignals=Body.BdyFrm.Cg.Vel.xdot,Driveline.EngSpd,Driveline.EMSpd,Engine.EngTrq,ElecMachine.EMTrq,Battery.BattCurr,Battery.BattSoc,Engine.EngineInfo.Afr,Engine.EngineInfo.FuelVolFlw,Battery.BattPwr
  Bus Selector3 : BusSelector  OutputSignals=LngRef
  Mux : Mux  Inputs=2
  Performance Calculations : Subsystem
  Rate Transition{1..2,4..5,7..8,10} (7 alike) : RateTransition  Deterministic=off
  Signal Specification3 : SignalSpecification  Unit=mph
  Signal Specification4 : SignalSpecification  Unit=rpm
  Signal Specification5 : SignalSpecification  Unit=rpm
  Signal Specification6 : SignalSpecification  Unit=mph
  Signal Specification7 : SignalSpecification  Unit=m/s
  Signal Specification8 : SignalSpecification  Unit=rad/s
  Signal Specification9 : SignalSpecification  Unit=rad/s
  Terminator4 : Terminator
  Terminator5 : Terminator
  Unit Conversion{,4..6} (4 alike) : UnitConversion
  "Trace Velocity, Target, Actual (mph)" : Outport
  EngSpd (RPM) : Outport  Port=2
  Engine Torque (Nm) : Outport  Port=3
  Electric Motor Speed (RPM) : Outport  Port=4
  Electric Motor Torque (Nm) : Outport  Port=5
  Battery Current (A) : Outport  Port=6
  Battery SOC : Outport  Port=7
  US Fuel Economy MPGe : Outport  Port=8
  wires:
  Signal Specification4/1 -> Rate Transition2/1
  Performance Calculations/2(L/100Km) -> Terminator4/1
  Bus Selector1/4 -> Rate Transition7/1  "<EngTrq>"
  Bus Selector1/7 -> Rate Transition1/1  "<BattSoc>"
  Signal Specification6/1 -> [VehSpd], Mux/2
  Bus Selector1/9 -> Performance Calculations/2(FuelVolFlow)  "<FuelVolFlw>"
  Bus Selector1/5 -> Rate Transition8/1  "<EMTrq>"
  Unit Conversion/1 -> Signal Specification3/1
  Bus Selector3/1 -> Signal Specification7/1  "<LngRef>"
  Bus Selector1/10 -> Performance Calculations/3(BattPwr)  "<BattPwr>"
  Bus Selector1/2 -> Signal Specification8/1  "<EngSpd>"
  Rate Transition7/1 -> Engine Torque (Nm)/1  "Engine Torque (Nm)"
  Mux/1 -> Rate Transition4/1
  Unit Conversion6/1 -> Signal Specification6/1
  Bus Selector1/6 -> Rate Transition10/1  "<BattCurr>"
  Signal Specification5/1 -> Rate Transition5/1
  Ref/1 -> Bus Selector3/1
  Signal Specification3/1 -> Mux/1
  Unit Conversion5/1 -> Signal Specification5/1
  Unit Conversion4/1 -> Signal Specification4/1
  Signal Specification9/1 -> Unit Conversion5/1
  Signal Specification8/1 -> Unit Conversion4/1
  Bus Selector1/8 -> Terminator5/1  "<Afr>"
  Rate Transition2/1 -> EngSpd (RPM)/1  "EngSpd (RPM)"
  Bus Selector1/3 -> Signal Specification9/1  "<EMSpd>"
  [VehSpd] -> Performance Calculations/1(VehSpd)
  Signal Specification7/1 -> Unit Conversion/1
  Bus Selector1/1 -> Unit Conversion6/1  "<xdot>"
  Rate Transition8/1 -> Electric Motor Torque (Nm)/1  "Electric Motor Torque (Nm)"
  Rate Transition4/1 -> "Trace Velocity, Target, Actual (mph)"/1  "Trace Velocity, Target, Actual (mph)"
  Rate Transition5/1 -> Electric Motor Speed (RPM)/1  "Electric Motor Speed (RPM)"
  VehFdbk/1 -> Bus Selector1/1
  Rate Transition1/1 -> Battery SOC/1  "Battery SOC"
  Rate Transition10/1 -> Battery Current (A)/1  "Battery Current (A)"
  Performance Calculations/1(US MPG) -> US Fuel Economy MPGe/1  "US Fuel Economy MPGe"

== system VirtualMotoTemplate/Visualization/Scope Type ==
  "Vis " : Inport
  "VehFdbk " : Inport  Port=2
  DLC : Subsystem  VariantControl=1
  None : Subsystem  VariantControl=0
  XYZ : Subsystem  VariantControl=2
  " Ref" : Outport  VectorParamsAs1DForOutWhenUnconnected=off

== system VirtualMotoTemplate/Visualization/Vehicle XY Plotter ==
  "Ref " : Inport
  "VehFdbk " : Inport  Port=2
  Disabled : Subsystem  VariantControl=2
  XY View : Subsystem  VariantControl=0
  XY View Ref : Subsystem  VariantControl=1

== system VirtualMotoTemplate/Environment/Friction/Constant Friction ==
  Friction Scaling : Constant  Value=ones(2,1).*EnvNomFrictionScaling  SampleTime=0
  FricCoeffLambda : Outport
  wires:
  Friction Scaling/1 -> FricCoeffLambda/1

== system VirtualMotoTemplate/Environment/Friction/Varying Friction ==
  MotoFdbk : Inport
  Bus Selector1 : BusSelector  OutputSignals=Whl.Genrl.Frnt.Cp.Disp.x,Whl.Genrl.Rear.Cp.Disp.x,Whl.Genrl.Frnt.Cp.Disp.y,Whl.Genrl.Rear.Cp.Disp.y
  Bus Selector2 : BusSelector  OutputSignals=Body.InertFrm.Cg.Disp
  Road Track Friction : Subsystem  mask(Road Track Friction){surface_popup=Split friction coefficient scaling factor, lambda_g=EnvNomFrictionScaling, lambda_r=.6, r_x0=175, r_y0=-100, r_xw=1000, r_yw=500, aMode=2}
      mask prompts: surface_popup "vdynblks:vehdynManFriction:blkPrm_surface_popup"; lambda_g "vdynblks:vehdynManFriction:blkPrm_lambda_g"; lambda_r "vdynblks:vehdynManFriction:blkPrm_lambda_r"; r_x0 "vdynblks:vehdynManFriction:blkPrm_r_x0"; r_y0 "vdynblks:vehdynManFriction:blkPrm_r_y0"; r_xw "vdynblks:vehdynManFriction:blkPrm_r_xw"; r_yw "vdynblks:vehdynManFriction:blkPrm_r_yw"
      mask init:
      | % Scaling factor for the friction coefficient around the rectangular region
      | mutable = [lambda_g, lambda_g, lambda_g, lambda_g;
      |            lambda_g, lambda_r, lambda_r, lambda_g; 
      |            lambda_g, lambda_r, lambda_r, lambda_g; 
      |            lambda_g, lambda_g, lambda_g, lambda_g ];
      |        
      | 
      | % The step is distance between breakpoint near the boundary of high and
      | % low friction coefficient
      | 
      | step = 0.01 ; 
      | 
      | % In the mask initialization, xbr and ybr breakpoints are with respect to
      | % Body fixed coordinate system. At time t=0, xbr and ybr breakpoints
      | % updates to Earth (Inertial) Fixed coordinate system. The breakpoints for
      | % the lookup table are added via inputs.
      | 
      | xbr = [(r_x0 - step) , (r_x0 + step), (r_x0 + r_xw - step) , (r_x0 + r_xw + step) ];
      | ybr = [(r_y0 - step) , (r_y0 + step), (r_y0 + r_yw - step) , (r_y0 + r_yw + step) ];
      | 
      | 
      | % To check if the created track is split mu or constant mu
      | 
      | surface_popup = get_param(gcb, 'surface_popup');
      | 
      | if strcmp(surface_popup, 'Split friction coefficient scaling factor')
      |     SplitLambdaTrck = 1;
      | elseif strcmp(surface_popup, 'Constant friction coefficient scaling factor')
      |     SplitLambdaTrck = 0;
      | end
      mask Help: eval('vdynblkshelp(''vdynblkstrack'')');
      mask TypeOptions surface_popup: vdynblks:vehdynManFriction:blkCmb_surface_popup_c1 | vdynblks:vehdynManFriction:blkCmb_surface_popup_c2
      mask Callback surface_popup:
      | surface_popup = get_param(gcb, 'surface_popup');
      | m = Simulink.Mask.get(gcb);
      | 
      | lambda_g = m.getParameter('lambda_g');
      | lambda_r = m.getParameter('lambda_r');
      | r_x0 = m.getParameter('r_x0');
      | r_y0 = m.getParameter('r_y0');
      | r_xw = m.getParameter('r_xw');
      | r_yw = m.getParameter('r_yw');
      | %track_view = m.getParameter('track_view');
      | 
      | 
      | if strcmp(surface_popup, 'Split friction coefficient scaling factor')
      |     lambda_g.Visible = 'on';
      |     lambda_r.Visible = 'on';
      |     r_x0.Visible = 'on';
      |     r_y0.Visible = 'on';
      |     r_xw.Visible = 'on';
      |     r_yw.Visible = 'on';
      |     %track_view.Visible = 'on';
      | 
      | elseif strcmp(surface_popup,'Constant friction coefficient scaling factor')
      |     lambda_g.Visible = 'on';
      |     lambda_r.Visible = 'off';
      |     r_x0.Visible = 'off';
      |     r_y0.Visible = 'off';
      |     r_xw.Visible = 'off';
      |     r_yw.Visible = 'off';
      |     %track_view.Visible = 'off';
      | end
      | [~]=autosharedicon('autolibutils',gcb,0);
      mask DialogControl DescGroupVar Prompt: Road Track Friction
      mask DialogControl DescTextVar Prompt: vdynblks:vehdynManFriction:blkDesc
      mask DialogControl surface_popup Prompt: Type of surface:
      mask DialogControl lambda_g Prompt: Scaling factor for the friction coefficient of ground, lambda_g :
      mask DialogControl lambda_r Prompt: Scaling factor for the friction coefficient of rectangular surface, lambda_r :
      mask DialogControl r_x0 Prompt: X coordinate of lower left corner of rectangular surface, r_x0 [m]:
      mask DialogControl r_y0 Prompt: Y coordinate of lower left corner of rectangular surface, r_y0 [m]:
      mask DialogControl r_xw Prompt: Rectangular surface width in X direction, r_xw [m]:
      mask DialogControl r_yw Prompt: Rectangular surface width in Y direction, r_yw [m]:
  Wheel Coordinates : Subsystem
  FricCoeffLambda : Outport
  wires:
  Wheel Coordinates/1(XWhl) -> Road Track Friction/1(XWhl)
  MotoFdbk/1 -> Bus Selector2/1, Bus Selector1/1
  Wheel Coordinates/2(YWhl) -> Road Track Friction/2(YWhl)
  Road Track Friction/1(FricCoeffLambda) -> FricCoeffLambda/1
  Bus Selector2/1 -> Road Track Friction/3(Cg)  "<Disp>"
  Bus Selector1/1 -> Wheel Coordinates/1(FrntAxlX)  "<x>"
  Bus Selector1/2 -> Wheel Coordinates/2(RearAxlX)  "<x>"
  Bus Selector1/3 -> Wheel Coordinates/3(FrntAxlY)  "<y>"
  Bus Selector1/4 -> Wheel Coordinates/4(RearAxlY)  "<y>"

== system VirtualMotoTemplate/Environment/Ground Feedback/3D Engine ==
  Friction : Inport
  WheelFdbk : Inport  Port=2
  3D Engine Source : Subsystem  Variant=on  VariantControl=Choice  mask(Terrain Source){terrType=Single point}
      mask prompts: terrType "Terrain feedback type:"
      mask help:
      | This variant subsystem provides the option for:
      | - a single point of contact for each wheel with minimal post-processing ideal for smooth surfaces and maximum run-time performance.
      | - multiple points of contact per wheel which may be used when interested in non-smooth terrain at a higher computational cost and requires Vehicle Dynamics Blockset.
      mask TypeOptions terrType: Single point | Multiple points
  Bus Creator2 : BusCreator  Inputs=2
  Bus Creator3 : BusCreator  Inputs=3
  Demux1 : Demux  Outputs=2
  Signal Specification1 : SignalSpecification  Unit=1
  Ground : Outport  VectorParamsAs1DForOutWhenUnconnected=off
  wires:
  3D Engine Source/2(DCM) -> Bus Creator3/2  "DCM"
  3D Engine Source/1(z) -> Bus Creator3/1  "z"
  WheelFdbk/1 -> 3D Engine Source/1(WheelFdbk)
  Friction/1 -> Signal Specification1/1
  Bus Creator3/1 -> Ground/1
  Bus Creator2/1 -> Bus Creator3/3  "mu"
  Demux1/2 -> Bus Creator2/2  "mu_R"
  Demux1/1 -> Bus Creator2/1  "mu_F"
  Signal Specification1/1 -> Demux1/1

== system VirtualMotoTemplate/Environment/Ground Feedback/Constant ==
  Friction : Inport
  Bus Creator : BusCreator  Inputs=2
  Bus Creator2 : BusCreator  Inputs=2
  Bus Creator3 : BusCreator  Inputs=3
  Constant1 : Constant  Value=zeros(2,1)
  Constant2 : Constant  Value=repmat(eye(3),1,1,2)  SampleTime=-1
  Demux : Demux  Outputs=2
  Demux1 : Demux  Outputs=2
  Signal Specification : SignalSpecification  Unit=m
  Signal Specification1 : SignalSpecification  Unit=1
  Ground : Outport  VectorParamsAs1DForOutWhenUnconnected=off
  wires:
  Constant1/1 -> Signal Specification/1
  Signal Specification/1 -> Demux/1
  Demux/1 -> Bus Creator/1  "G_F_z"
  Demux/2 -> Bus Creator/2  "G_R_z"
  Bus Creator/1 -> Bus Creator3/1  "z"
  Demux1/1 -> Bus Creator2/1  "mu_F"
  Demux1/2 -> Bus Creator2/2  "mu_R"
  Bus Creator2/1 -> Bus Creator3/3  "mu"
  Friction/1 -> Signal Specification1/1
  Signal Specification1/1 -> Demux1/1
  Bus Creator3/1 -> Ground/1
  Constant2/1 -> Bus Creator3/2  "DCM"

== system VirtualMotoTemplate/Motorcycle Vehicle/Body, Steer, Suspension, Wheels/Body, Steer, Suspension, Wheels ==
  WindXYZ : Inport
  BrkPrs : Inport  Port=2
  MDrvSprtR : Inport  Port=3
  MDrvArmR : Inport  Port=4
  MDrvFrm : Inport  Port=5
  ScaleFactrs : Inport  Port=6
  SteerCmd : Inport  Port=7
  In_Plane_Model : Subsystem  VariantControl=In_Plane_Model  ReferencedSubsystem=In_Plane_Model
  Out_of_Plane_Model : Subsystem  VariantControl=Out_of_Plane_Model  ReferencedSubsystem=Out_of_Plane_Model
  Moto : Outport
  Wheels : Outport  Port=2

== system VirtualMotoTemplate/Motorcycle Vehicle/Body, Steer, Suspension, Wheels/Chassis Input ==
  Env : Inport
  Driveline : Inport  Port=2
  Rider : Inport  Port=3
  Bus Selector : BusSelector  OutputSignals=SteerFdbk
  Bus Selector2 : BusSelector  OutputSignals=Wind,Gnd.mu
  Bus Selector4 : BusSelector  OutputSignals=BrkPrs,Info.ChainInfo.MDrvSprtR,Info.MDrvArmR,Info.MDrvFrm
  Bus to Vector : BusToVector
  Wind : Outport  VectorParamsAs1DForOutWhenUnconnected=off
  BrkPrs : Outport  Port=2  VectorParamsAs1DForOutWhenUnconnected=off
  MDrvSprtR : Outport  Port=3  VectorParamsAs1DForOutWhenUnconnected=off
  MDrvArmR : Outport  Port=4  VectorParamsAs1DForOutWhenUnconnected=off
  MDrvFrm : Outport  Port=5  VectorParamsAs1DForOutWhenUnconnected=off
  ScaleFactrs : Outport  Port=6  VectorParamsAs1DForOutWhenUnconnected=off
  SteerCmd : Outport  Port=7  VectorParamsAs1DForOutWhenUnconnected=off
  wires:
  Env/1 -> Bus Selector2/1
  Bus Selector2/1 -> Wind/1  "<Wind>"
  Driveline/1 -> Bus Selector4/1
  Bus Selector4/4 -> MDrvFrm/1  "<MDrvFrm>"
  Bus Selector4/3 -> MDrvArmR/1  "<MDrvArmR>"
  Bus Selector4/2 -> MDrvSprtR/1  "<MDrvSprtR>"
  Bus Selector4/1 -> BrkPrs/1  "<BrkPrs>"
  Bus Selector2/2 -> Bus to Vector/1  "<mu>"
  Bus to Vector/1 -> ScaleFactrs/1
  Rider/1 -> Bus Selector/1
  Bus Selector/1 -> SteerCmd/1  "<SteerFdbk>"

== system VirtualMotoTemplate/Motorcycle Vehicle/Body, Steer, Suspension, Wheels/Chassis Output ==
  Moto : Inport
  Wheels : Inport  Port=2
  Out Bus Element4 : Outport  PortName=MotoFdbk
  Out Bus Element1 : Outport  Port=2  PortName=WheelsFdbk
  wires:
  Moto/1 -> Out Bus Element4/1
  Wheels/1 -> Out Bus Element1/1

== system VirtualMotoTemplate/Motorcycle Vehicle/Control Feedback/Variant Subsystem ==
  note: 1) Add Subsystem or Model blocks as valid variant choices.
      | 2) You cannot connect blocks at this level. At simulation, connectivity is automatically
      | determined, based on the active variant and port name matching.
  MotoFdbk : Inport
  IMU_Sensor : Subsystem  VariantControl=IMU_Sensor  ReferencedSubsystem=IMU_Sensor
  No_IMU_Sensor : Subsystem  VariantControl=No_IMU_Sensor  ReferencedSubsystem=No_IMU_Sensor
  IMU : Outport

== system VirtualMotoTemplate/Motorcycle Vehicle/Hand Levers and Pedals/Hand Levers and Pedals ==
  note: Placeholder for introducing faults, detailed actuator behavior,
      | interactions of other systems with a human interface such
      | as changes in power steering and braking assistance.
  SteerCmd : Inport
  AccCmd : Inport  Port=2
  DecelCmd : Inport  Port=3
  GearCmd : Inport  Port=4
  BrkPrs : Inport  Port=5
  StrWhlTrq : Inport  Port=6
  Brake Pedal : Subsystem
  Dead Zone3 : DeadZone  LowerValue=-.01  UpperValue=.01  ZeroCross=off
  Terminator : Terminator
  Terminator1 : Terminator
  Twist2Acc : Lookup_n-D  NumberOfTableDimensions=1  BreakpointsForDimension1=[0 1]  Table=[0 1]  ExtrapMethod=Clip  InternalRulePriority=Speed  RndMeth=Simplest
  SteerFdbk : Outport
  AccFdbk : Outport  Port=2
  DecelFdbk : Outport  Port=3
  GearFdbk : Outport  Port=4
  wires:
  SteerCmd/1 -> Dead Zone3/1
  DecelCmd/1 -> Brake Pedal/1(DecelCmd)
  GearCmd/1 -> GearFdbk/1
  BrkPrs/1 -> Terminator/1
  StrWhlTrq/1 -> Terminator1/1
  Brake Pedal/1(DecelFdbk) -> DecelFdbk/1
  Dead Zone3/1 -> SteerFdbk/1
  AccCmd/1 -> Twist2Acc/1
  Twist2Acc/1 -> AccFdbk/1

== system VirtualMotoTemplate/Motorcycle Vehicle/Hand Levers and Pedals/Pedal Cluster Input ==
  Rider : Inport
  Driveline : Inport  Port=2
  Bus Selector : BusSelector  OutputSignals=SteerCmd,AccelCmd,DecelCmd,GearCmd
  Bus Selector1 : BusSelector  OutputSignals=EMSpd
  Constant : Constant  Value=0
  SteerCmd : Outport  VectorParamsAs1DForOutWhenUnconnected=off
  AccelCmd : Outport  Port=2  VectorParamsAs1DForOutWhenUnconnected=off
  DecelCmd : Outport  Port=3  VectorParamsAs1DForOutWhenUnconnected=off
  GearCmd : Outport  Port=4  VectorParamsAs1DForOutWhenUnconnected=off
  BrkPrs : Outport  Port=5  VectorParamsAs1DForOutWhenUnconnected=off
  StrWhlTrq : Outport  Port=6  VectorParamsAs1DForOutWhenUnconnected=off
  wires:
  Bus Selector/2 -> AccelCmd/1  "<AccelCmd>"
  Rider/1 -> Bus Selector/1
  Bus Selector/3 -> DecelCmd/1  "<DecelCmd>"
  Bus Selector/4 -> GearCmd/1  "<GearCmd>"
  Bus Selector/1 -> SteerCmd/1  "<SteerCmd>"
  Driveline/1 -> Bus Selector1/1
  Bus Selector1/1 -> BrkPrs/1  "<EMSpd>"
  Constant/1 -> StrWhlTrq/1

== system VirtualMotoTemplate/Motorcycle Vehicle/Hand Levers and Pedals/Pedal Cluster Output ==
  SteerFdbk : Inport
  AccFdbk : Inport  Port=2
  DecelFdbk : Inport  Port=3
  GearFdbk : Inport  Port=4
  Bus Creator1 : BusCreator  Inputs=4
  Signal Specification : SignalSpecification  Unit=N*m
  Signal Specification1 : SignalSpecification  Unit=1
  Signal Specification2 : SignalSpecification  Unit=1
  Signal Specification3 : SignalSpecification  Unit=1
  OperatorFdbk : Outport
  wires:
  Signal Specification1/1 -> Bus Creator1/2  "AccFdbk"
  Signal Specification3/1 -> Bus Creator1/4  "GearFdbk"
  AccFdbk/1 -> Signal Specification1/1
  DecelFdbk/1 -> Signal Specification2/1
  GearFdbk/1 -> Signal Specification3/1
  Signal Specification/1 -> Bus Creator1/1  "SteerFdbk"
  SteerFdbk/1 -> Signal Specification/1
  Bus Creator1/1 -> OperatorFdbk/1
  Signal Specification2/1 -> Bus Creator1/3  "DecelFdbk"
